simulink model "H8_6GDL_nolineal_desactualizado"  (R2022b)
settings: Solver=VariableStepAuto  StartTime=0.0  StopTime=3  MaxStep=1e-3  RelTol=1e-3
InitFcn:
  | %load("ems.mat");
  | %load("hems.mat");
  | %load("Ka.mat");
  | load('fuerzasY_LIM.mat')
  | load('matrices_linealizacion_6gdl.mat')
  | m = 200;
  | g = 9.81;
  | 
  | x_lev12 = 0.443;
  | x_lev34 = 0.542;%0.443;
  | x_guid12 = 0.4475;
  | x_guid34 = 0.5465;
  | x_lim = 0.0495;
  | 
  | y_lev13 = 0.23686;
  | y_lev24 = 0.23686;
  | y_guid13 = 0.24263;
  | y_guid24 = 0.24263;
  | y_lim = 0.0005;
  | y_brk = 0.21552;
  | 
  | z_lev = 0.08546;
  | z_guid = 0.026;
  | z_lim = 0.1055;
  | z_brk = 0.03941;
  | 
  | kp_lev = 50;
  | ki_lev = 400;
  | kp_guid = 6;
  | ki_guid = 46.5;
  | 
  | Imax_lev = 50;
  | Imin_lev = -50;
  | Imax_guid = 50;
  | Imin_guid = 0;
  | 
  | cg_nom=0.567;
  | lev_nom=0.01965;
  | cg_suelo=0.56985;
  | cg_techo=0.55735;
  | 
  | I = [43.082 0 0; 0 26.887 -0; 0 0 29.297]
values from neighbouring files (symbols this model uses):
  A6 = [0 0 0 0 0 0 0 0 0 0 0 0 ... (100 elements, 10x10)]    [matrices_linealizacion_6gdl.mat]
  B6 = [0 0 0 0 0 0.000575563603666 -0.0459993641186 -0.0505103975277 0.151580453785 0.00175830093621 0 0 ... (80 elements, 10x8)]    [matrices_linealizacion_6gdl.mat]
  C6 = [1 0 0 0 0 0 0 0 0 0 0 1 ... (100 elements, 10x10)]    [matrices_linealizacion_6gdl.mat]
  current = [0 10 20 30 40 50 60 70 80 90 100]    [fuerzasY_LIM.mat]
  D6 = [0 0 0 0 0 0 0 0 0 0 0 0 ... (80 elements, 10x8)]    [matrices_linealizacion_6gdl.mat]
  Ka = [34.5916764023 4.46928641015 34.7816336405 4.65924364837 92.2484067139 -92.2484067139 74.2332308826 -74.2332308826 -4220.94514487 -4209.6309051 -4205.06787146 -4193.7536317 ... (120 elements, 8x15)]    [Ka.mat]    (also in linealizacion_5gdl_bien.m = place(Aa,Ba,[ -1.5 -1.5 -1.5 -1.5 -2 -2 -6 -6 -7 -7 -5 -5 -2; linealizacion_EMS.m = place(Aa,Ba,[ -1 -1 -2 -2 -3 -3 -6 -6 -7 -7 -5 -5 -4 -4 -5 -)
  Y = [0 1 2 3 4 5 6]    [fuerzasY_LIM.mat]
undefined symbols (not defined in the file or in its folder): ems, FuerzaRail_Y, hems, magnitude
libraries: slpidlib x16
(part 1 of 2)
settings Model: Creator=USUARIO  LastModifiedBy=USUARIO
settings SolverCC: ZeroCrossAlgorithm=Adaptive

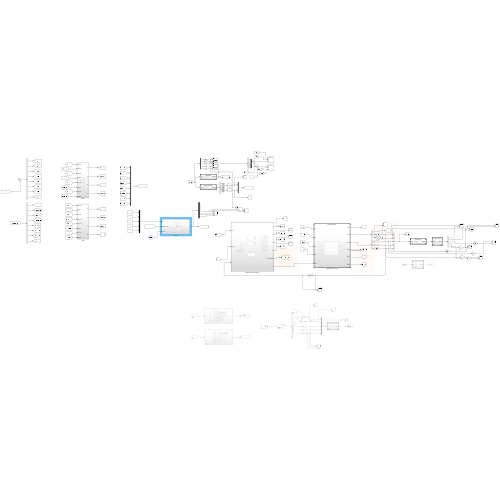
[thumbnail: Simulink's stored preview of the top-level diagram]
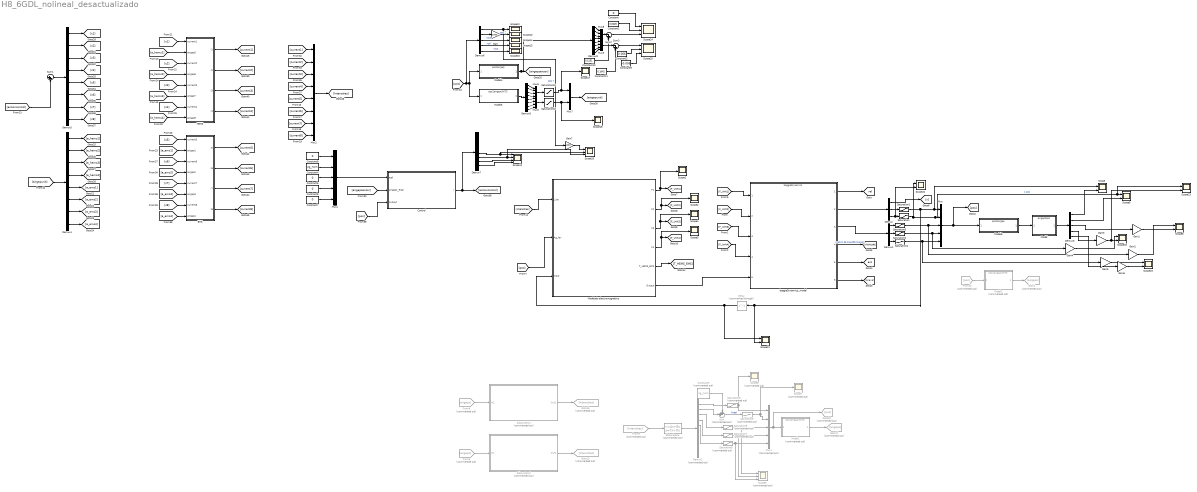
== system H8_6GDL_nolineal_desactualizado ==
  Constant{,5..8} (5 alike) : Constant  Value=0
  Constant1 : Constant  Value=0.0225
  Constant10 : Constant  Value=0.1251
  Constant11 : Constant  Value=0.1042
  Constant2 : Constant  Value=0.006
  Constant3 : Constant  Commented=on  Value=cg_nom
  Constant4 : Constant  Value=cg_nom
  Constant9 : Constant  Value=-0.006
  Control : Subsystem
  Delay : Delay  Commented=through  DelayLength=1  InitialCondition=0.001
  Demux : Demux  Outputs=3
  Demux1 : Demux  Outputs=3
  Demux2 : Demux  Commented=on  Outputs=10
      settings: DisplayOption=none
  Demux3 : Demux  Outputs=5
  Demux{4..5,7..9} (5 alike) : Demux  Outputs=8
  Demux6 : Demux  Outputs=5
  EMS : Subsystem
  From40 : From  Commented=on  GotoTag=pos
  From6 : From  Commented=on  GotoTag=airgaps
  From8 : From  Commented=on  GotoTag=airgaps
  From9 : From  Commented=on  GotoTag=Intensities
  Gain : Gain  Gain=1000
  Gain{1..6} (6 alike) : Gain  Gain=180/pi
  Gain7 : Gain  Gain=1000
  Goto1 : Goto  Commented=on  GotoTag=airgaps
  Goto13 : Goto  Commented=on  GotoTag=Intensities
  Goto16 : Goto  Commented=on  GotoTag=Intensities
  Goto17 : Goto  Commented=on  GotoTag=airgaps
  Goto18 : Goto  Commented=on  GotoTag=pos
  HEMS : Subsystem
  Model : ModelReference  ModelNameDialog=airgap2pos.slx  SimulationMode=Normal  ModelReferenceVersion=1.7
  Model1 : ModelReference  Commented=on  ModelNameDialog=pos2airgapUNITS.slx  SimulationMode=Normal  ModelReferenceVersion=1.3
  Model2 : ModelReference  Commented=on  ModelNameDialog=pos2airgapUNITS.slx  SimulationMode=Normal  ModelReferenceVersion=1.3
  Model4 : ModelReference  ModelNameDialog=pos2airgap.slx  SimulationMode=Normal  ModelReferenceVersion=1.6
  Model5 : ModelReference  ModelNameDialog=pos2airgapUNITS.slx  SimulationMode=Normal  ModelReferenceVersion=1.3
  Model6 : ModelReference  ModelNameDialog=pos2airgap.slx  SimulationMode=Normal  ModelReferenceVersion=1.6
  Modelado electromagnetico : Subsystem
  Mux : Mux  Inputs=5
  Mux1 : Mux  Commented=on  Inputs=5
  Mux2 : Mux  Inputs=8
  Mux{3,5..6,8} (4 alike) : Mux
  Mux4 : Mux  Inputs=5
  Mux7 : Mux  Inputs=2
  Saturation : Saturate  UpperLimit=cg_suelo  LowerLimit=cg_techo
  Saturation1 : Saturate  UpperLimit=0.012  LowerLimit=-0.012
  Saturation15 : Saturate  UpperLimit=0.0225  LowerLimit=0.01
  Saturation16 : Saturate  UpperLimit=0.024  LowerLimit=0
  Saturation2 : Saturate  UpperLimit=0.01268  LowerLimit=-0.01268
  Saturation3 : Saturate  UpperLimit=0.0476  LowerLimit=-0.0476
  Saturation4 : Saturate  UpperLimit=0.024  LowerLimit=-0.024
  Saturation5 : Saturate  Commented=on  UpperLimit=cg_suelo  LowerLimit=cg_techo
  Saturation6 : Saturate  Commented=on  UpperLimit=0.012  LowerLimit=-0.012
  Saturation7 : Saturate  Commented=on  UpperLimit=0.01268  LowerLimit=-0.01268
  Saturation8 : Saturate  Commented=on  UpperLimit=0.0476  LowerLimit=-0.0476
  Saturation9 : Saturate  Commented=on  UpperLimit=0.024  LowerLimit=-0.024
  Scope{,5..6,18..19,21..23} (8 alike) : Scope  NumInputPorts=2
  Scope{1..4,10,12..17} (11 alike) : Scope
  Scope11 : Scope  NumInputPorts=4
  Scope20 : Scope  NumInputPorts=3
  Scope24 : Scope  NumInputPorts=3
  Scope25 : Scope  NumInputPorts=3
  Scope7 : Scope  Commented=on
  Scope8 : Scope  Commented=on
  Scope9 : Scope  Commented=on  NumInputPorts=3
  State-Space : StateSpace  Commented=on  A=A6  B=B6  C=C6  D=D6  InitialCondition=[-0.001 0.001 0.001 -0.001 0.001 0 0 0 0 0]
  Subsystem1 : Subsystem  Commented=on
  Subsystem2 : Subsystem  Commented=on
  Sum : Sum  Commented=on  Inputs=++|
  Sum1 : Sum  Inputs=|+-
  Sum2 : Sum  Inputs=|-+
  Sum3 : Sum  Inputs=|-+
  boggieDynamics_model : ModelReference  ModelNameDialog=boggieDynamics.mdl  SimulationMode=Normal  ModelReferenceVersion=1.35
  tag scope: acc=global, vel=global
  wires:
  [F_Unit4] -> boggieDynamics_model/4
  [F_Unit3] -> boggieDynamics_model/3
  [F_Unit2] -> boggieDynamics_model/2
  boggieDynamics_model/4 -> [Attitude]  "matriz de transformacion"
  [F_Unit1] -> boggieDynamics_model/1
  boggieDynamics_model/3 -> Demux1/1
  Mux/1 -> Model6/1, [pos]
  boggieDynamics_model/2 -> Demux/1
  Demux/3 -> Scope22/2, Saturation/1
  Demux/1 -> [x]
  boggieDynamics_model/1 -> [vel]
  Demux/2 -> Saturation1/1
  boggieDynamics_model/5 -> [acc]
  boggieDynamics_model/6 -> [angvel]
  [pos] -> Modelado electromagnetico/2(Ag_lev)
  [Intensities] -> Modelado electromagnetico/1(I_lev)
  Modelado electromagnetico/3(F3) -> Scope4/1, [F_Unit3]
  Modelado electromagnetico/2(F2) -> Scope2/1, [F_Unit2]
  Modelado electromagnetico/1(F1) -> Scope1/1, [F_Unit1]
  Modelado electromagnetico/5(T_HEMS_EMS) -> [T_HEMS_EMS]
  Demux1/1 -> Saturation3/1
  Demux1/2 -> Saturation2/1
  Demux1/3 -> Saturation4/1
  Model2/1 -> Goto1/1
  Saturation1/1 -> Scope21/2, Delay/1, Scope/1, Mux/1
  Saturation/1 -> Scope22/1, Scope23/1, Scope5/1, Mux/2  "z pos"
  Saturation3/1 -> Gain2/1, Mux/3
  Saturation2/1 -> Gain4/1, Mux/4
  Saturation4/1 -> Gain5/1, Mux/5
  Modelado electromagnetico/4(F4) -> Scope3/1, [F_Unit4]
  Subsystem1/1(Out1) -> Goto16/1
  From8/1 -> Subsystem1/1(In1)
  From6/1 -> Subsystem2/1(In1)
  Subsystem2/1(Out1) -> Goto13/1
  From9/1 -> State-Space/1
  State-Space/1 -> Demux2/1
  Demux2/3 -> Saturation8/1
  Saturation7/1 -> Scope9/2, Mux1/4
  Saturation8/1 -> Mux1/3, Scope9/1
  Demux2/4 -> Saturation7/1
  Saturation9/1 -> Mux1/5, Scope9/3
  Model1/1 -> Goto17/1
  Demux2/5 -> Saturation9/1
  Saturation6/1 -> Mux1/1, Scope8/1
  Demux2/1 -> Saturation6/1
  Mux1/1 -> Model1/1, Goto18/1
  Constant3/1 -> Sum/1
  Demux2/2 -> Sum/2
  Sum/1 -> Saturation5/1  "lineal"
  Saturation5/1 -> Mux1/2, Scope7/1
  Demux4/5 -> [a_ems1]
  HEMS/2(I2) -> [current2]
  [a_hems1] -> HEMS/2(airgap5)
  Demux4/7 -> [a_ems3]
  [current8] -> Mux2/8
  Demux4/8 -> [a_ems4]
  Demux5/5 -> [c5]
  Demux4/6 -> [a_ems2]
  [accioncontrol] -> Sum1/2
  [airgapsensor] -> Control/2(airgaps_Real)
  Demux4/2 -> [a_hems2]
  Demux5/2 -> [c2]
  Demux5/4 -> [c4]
  Mux7/1 -> [airgapunit]
  Saturation16/1 -> Scope16/1, Mux7/2
  Saturation15/1 -> Scope17/1, Mux7/1
  Demux7/8 -> Scope11/4
  Mux5/1 -> Saturation16/1
  Demux8/6 -> Mux5/2
  Demux8/7 -> Mux5/3
  Mux6/1 -> Saturation15/1
  Demux8/3 -> Mux6/3
  Demux8/5 -> Mux5/1
  Demux5/3 -> [c3]
  Demux8/2 -> Mux6/2
  Sum1/1 -> Demux5/1
  [current5] -> Mux2/5
  Demux6/3 -> Scope14/1  "rotX"
  [current6] -> Mux2/6
  [current7] -> Mux2/7
  HEMS/1(I1) -> [current1]
  Demux7/5 -> Scope20/2, Scope11/1
  Constant5/1 -> Mux4/3
  [a_ems1] -> EMS/2(airgap1)
  Mux4/1 -> Control/1(Ref)
  [c8] -> EMS/7(current8)
  [c3] -> HEMS/5(current3)
  Demux6/5 -> Scope15/1  "rotZ"
  Demux5/1 -> [c1]
  [c5] -> EMS/1(current5)
  Demux7/6 -> Scope20/3, Scope11/2
  Constant6/1 -> Mux4/4
  [c2] -> HEMS/3(current2)
  [current1] -> Mux2/1
  [c1] -> HEMS/1(current1)
  [a_hems3] -> HEMS/6(airgap7)
  [a_ems3] -> EMS/6(airgap3)
  [a_hems4] -> HEMS/8(airgap8)
  Demux4/1 -> [a_hems1]
  [a_ems4] -> EMS/8(airgap4)
  [a_hems2] -> HEMS/4(airgap6)
  Demux5/7 -> [c7]
  [current3] -> Mux2/3
  Model4/1 -> Demux9/1, [airgapsensor]
  [c4] -> HEMS/7(current4)
  [c7] -> EMS/5(current7)
  Demux6/4 -> Scope13/1  "rotY"
  Demux7/7 -> Scope11/3
  Demux4/4 -> [a_hems4]
  EMS/4(I8) -> [current8]
  EMS/2(I6) -> [current6]
  Gain/1 -> Scope10/1  "pos Z"
  Constant4/1 -> Mux4/2
  Constant8/1 -> Mux4/1
  Demux5/6 -> [c6]
  Constant7/1 -> Mux4/5
  Demux4/3 -> [a_hems3]
  Demux8/8 -> Mux5/4
  Demux6/2 -> Gain/1
  EMS/3(I7) -> [current7]
  Demux8/1 -> Mux6/1
  [current2] -> Mux2/2
  [a_ems2] -> EMS/4(airgap2)
  [current4] -> Mux2/4
  Demux5/8 -> [c8]
  Mux2/1 -> [Intensities]
  Demux6/1 -> Gain7/1, Scope12/1  "pos Y"
  [c6] -> EMS/3(current6)
  Demux8/4 -> Mux6/4
  HEMS/3(I3) -> [current3]
  HEMS/4(I4) -> [current4]
  [airgapunit] -> Demux4/1
  EMS/1(I5) -> [current5]
  [pos] -> Demux6/1, Model4/1, Model5/1
  Model5/1 -> Demux8/1
  Control/1(I) -> Demux7/1, [accioncontrol]
  [pos] -> Control/3(Output)
  From40/1 -> Model2/1
  Model6/1 -> Model/1
  Model/1 -> Demux3/1
  Demux3/1 -> Scope/2
  Demux3/2 -> Scope5/2
  Demux3/3 -> Gain1/1
  Demux3/4 -> Gain3/1
  Demux3/5 -> Gain6/1
  Modelado electromagnetico/6(Output) -> boggieDynamics_model/5
  Delay/1 -> Scope21/1, Modelado electromagnetico/3(Input)
  Gain1/1 -> Scope6/2
  Gain2/1 -> Scope6/1
  Gain3/1 -> Scope23/2, Scope18/2
  Gain4/1 -> Scope18/1
  Gain5/1 -> Scope19/1
  Gain6/1 -> Scope19/2
  Gain7/1 -> Scope20/1
  Demux9/6 -> Mux3/2
  Demux9/8 -> Mux3/4
  Demux9/4 -> Mux8/4
  Demux9/7 -> Mux3/3
  Demux9/5 -> Mux3/1
  Demux9/3 -> Mux8/3
  Demux9/1 -> Mux8/1
  Mux3/1 -> Sum3/1
  Mux8/1 -> Sum2/1
  Demux9/2 -> Mux8/2
  Sum2/1 -> Scope24/3
  Constant1/1 -> Scope24/2
  Constant/1 -> Scope24/1
  Sum3/1 -> Scope25/1
  Constant9/1 -> Scope25/3
  Constant2/1 -> Scope25/2
  Constant10/1 -> Sum2/2
  Constant11/1 -> Sum3/2

== system H8_6GDL_nolineal_desactualizado/Control ==
  Ref : Inport
  airgaps_Real : Inport  Port=2
  Output : Inport  Port=3
  Demux : Demux  Outputs=5
  Demux1 : Demux  Outputs=5
  Model : ModelReference  ModelNameDialog=airgap2pos.slx  SimulationMode=Normal  ModelReferenceVersion=1.7
  Saturation4 : Saturate  Commented=through  UpperLimit=55  LowerLimit=-55
  Scope{,1..4} (5 alike) : Scope  NumInputPorts=2
  state space control : Subsystem
  I : Outport
  wires:
  airgaps_Real/1 -> Model/1
  Saturation4/1 -> I/1
  Model/1 -> Demux/1
  Ref/1 -> state space control/2(In2)
  state space control/1(Out1) -> Saturation4/1
  Demux/1 -> Scope1/1
  Demux/3 -> Scope/1
  Demux/4 -> Scope3/2
  Demux/2 -> Scope2/2
  Output/1 -> state space control/1(Output), Demux1/1
  Demux1/1 -> Scope1/2
  Demux1/2 -> Scope2/1
  Demux1/3 -> Scope/2
  Demux1/4 -> Scope3/1
  Demux1/5 -> Scope4/1
  Demux/5 -> Scope4/2

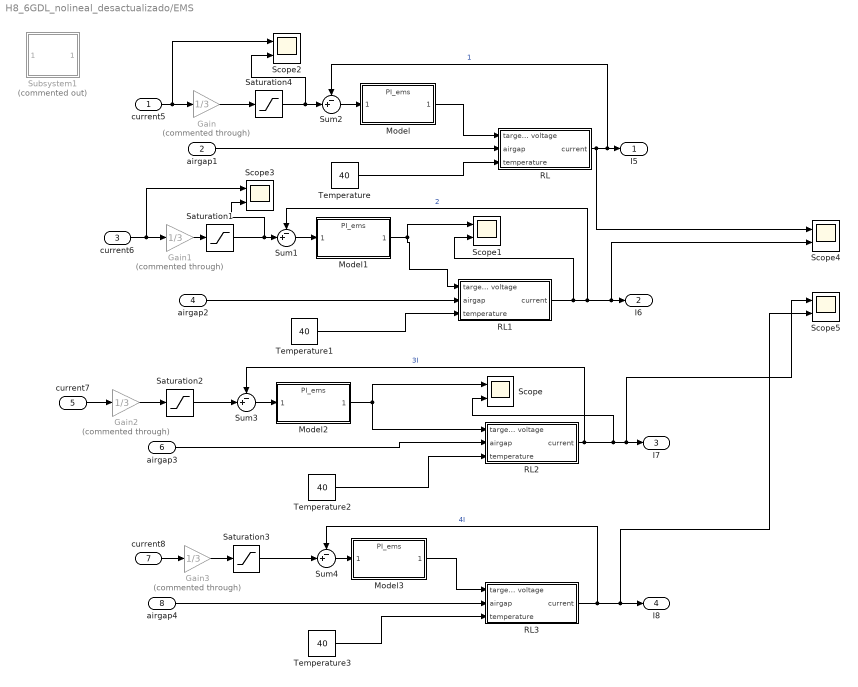
== system H8_6GDL_nolineal_desactualizado/EMS ==
  current5 : Inport
  airgap1 : Inport  Port=2
  current6 : Inport  Port=3
  airgap2 : Inport  Port=4
  current7 : Inport  Port=5
  airgap3 : Inport  Port=6
  current8 : Inport  Port=7
  airgap4 : Inport  Port=8
  Gain{,1..3} (4 alike) : Gain  Commented=through  Gain=1/3
  Model{,1..3} (4 alike) : ModelReference  ModelNameDialog=PI_ems.slx  SimulationMode=Normal  ModelReferenceVersion=1.2
  RL : Subsystem
  RL1 : Subsystem
  RL2 : Subsystem
  RL3 : Subsystem
  Saturation{1..4} (4 alike) : Saturate  UpperLimit=50  LowerLimit=0
  Scope{,1..5} (6 alike) : Scope  NumInputPorts=2
  Subsystem1 : Subsystem  Commented=on
  Sum{1..4} (4 alike) : Sum  Inputs=-+|
  Temperature{,1..3} (4 alike) : Constant  Value=40
  I5 : Outport
  I6 : Outport  Port=2
  I7 : Outport  Port=3
  I8 : Outport  Port=4
  wires:
  Temperature/1 -> RL/3(temperature)
  airgap1/1 -> RL/2(airgap)
  Temperature3/1 -> RL3/3(temperature)
  RL/1(current) -> Scope4/1, I5/1, Sum2/1  "1"
  current8/1 -> Gain3/1
  Temperature1/1 -> RL1/3(temperature)
  Temperature2/1 -> RL2/3(temperature)
  RL3/1(current) -> Scope5/2, I8/1, Sum4/1  "4I"
  current7/1 -> Gain2/1
  airgap2/1 -> RL1/2(airgap)
  RL1/1(current) -> Scope1/2, Scope4/2, I6/1, Sum1/1  "2"
  RL2/1(current) -> Scope/2, Scope5/1, I7/1, Sum3/1  "3I"
  airgap3/1 -> RL2/2(airgap)
  airgap4/1 -> RL3/2(airgap)
  Sum2/1 -> Model/1
  Sum1/1 -> Model1/1
  Sum3/1 -> Model2/1
  Sum4/1 -> Model3/1
  Model/1 -> RL/1(target voltage)
  Model3/1 -> RL3/1(target voltage)
  Model2/1 -> RL2/1(target voltage), Scope/1
  Model1/1 -> RL1/1(target voltage), Scope1/1
  current5/1 -> Scope2/1, Gain/1
  Saturation4/1 -> Scope2/2, Sum2/2
  Saturation1/1 -> Scope3/2, Sum1/2
  Saturation2/1 -> Sum3/2
  Saturation3/1 -> Sum4/2
  current6/1 -> Scope3/1, Gain1/1
  Gain/1 -> Saturation4/1
  Gain1/1 -> Saturation1/1
  Gain2/1 -> Saturation2/1
  Gain3/1 -> Saturation3/1

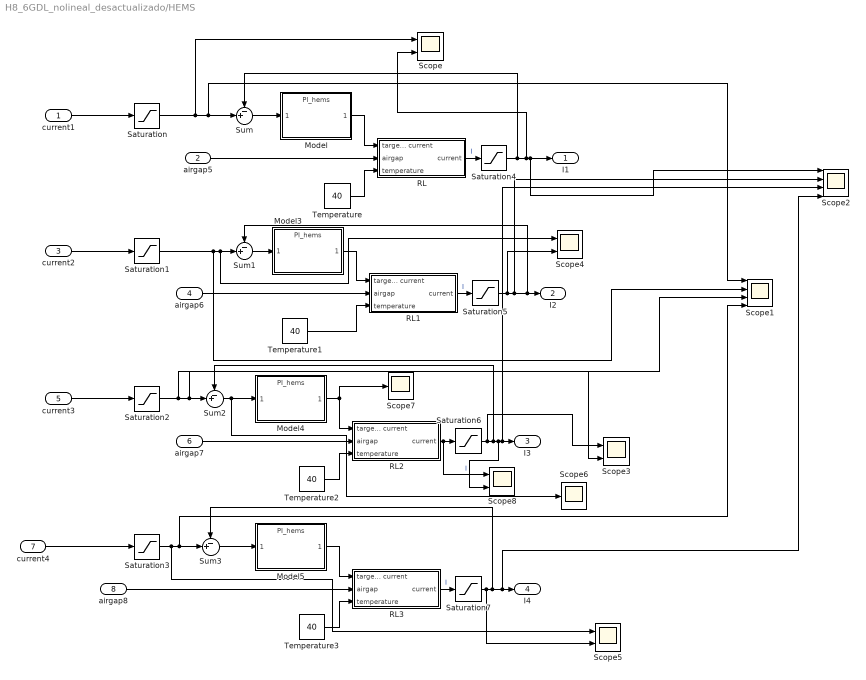
== system H8_6GDL_nolineal_desactualizado/HEMS ==
  current1 : Inport
  airgap5 : Inport  Port=2
  current2 : Inport  Port=3
  airgap6 : Inport  Port=4
  current3 : Inport  Port=5
  airgap7 : Inport  Port=6
  current4 : Inport  Port=7
  airgap8 : Inport  Port=8
  Model{,3..5} (4 alike) : ModelReference  ModelNameDialog=PI_hems.slx  SimulationMode=Normal  ModelReferenceVersion=1.3
  RL : Subsystem
  RL1 : Subsystem
  RL2 : Subsystem
  RL3 : Subsystem
  Saturation{,1..7} (8 alike) : Saturate  UpperLimit=50  LowerLimit=-50
  Scope{,3..5,8} (5 alike) : Scope  NumInputPorts=2
  Scope1 : Scope  NumInputPorts=4
  Scope2 : Scope  NumInputPorts=4
  Scope6 : Scope
  Scope7 : Scope
  Sum{,1..3} (4 alike) : Sum  Inputs=-+|
  Temperature{,1..3} (4 alike) : Constant  Value=40
  I1 : Outport
  I2 : Outport  Port=2
  I3 : Outport  Port=3
  I4 : Outport  Port=4
  wires:
  Temperature/1 -> RL/3(temperature)
  Model3/1 -> RL1/1(target current)
  Model5/1 -> RL3/1(target current)
  Model/1 -> RL/1(target current)
  airgap5/1 -> RL/2(airgap)
  Temperature3/1 -> RL3/3(temperature)
  RL/1(current) -> Saturation4/1  "I"
  Temperature1/1 -> RL1/3(temperature)
  Temperature2/1 -> RL2/3(temperature)
  Model4/1 -> RL2/1(target current), Scope7/1
  RL3/1(current) -> Saturation7/1  "I"
  airgap6/1 -> RL1/2(airgap)
  RL1/1(current) -> Saturation5/1  "I"
  RL2/1(current) -> Scope8/1, Saturation6/1  "I"
  airgap7/1 -> RL2/2(airgap)
  airgap8/1 -> RL3/2(airgap)
  Sum/1 -> Model/1
  Sum1/1 -> Model3/1
  Sum2/1 -> Scope6/1, Model4/1
  Sum3/1 -> Model5/1
  Saturation2/1 -> Scope3/2, Scope1/3, Sum2/2
  Saturation1/1 -> Scope1/2, Scope4/1, Sum1/2
  Saturation/1 -> Scope/1, Scope1/1, Sum/2
  Saturation3/1 -> Scope5/1, Scope1/4, Sum3/2
  current1/1 -> Saturation/1
  current4/1 -> Saturation3/1
  current3/1 -> Saturation2/1
  current2/1 -> Saturation1/1
  Saturation4/1 -> Scope/2, Scope2/1, I1/1, Sum/1
  Saturation5/1 -> Scope4/2, Scope2/2, Sum1/1, I2/1
  Saturation7/1 -> Scope5/2, Scope2/4, I4/1, Sum3/1
  Saturation6/1 -> Scope3/1, Scope8/2, Scope2/3, I3/1, Sum2/1

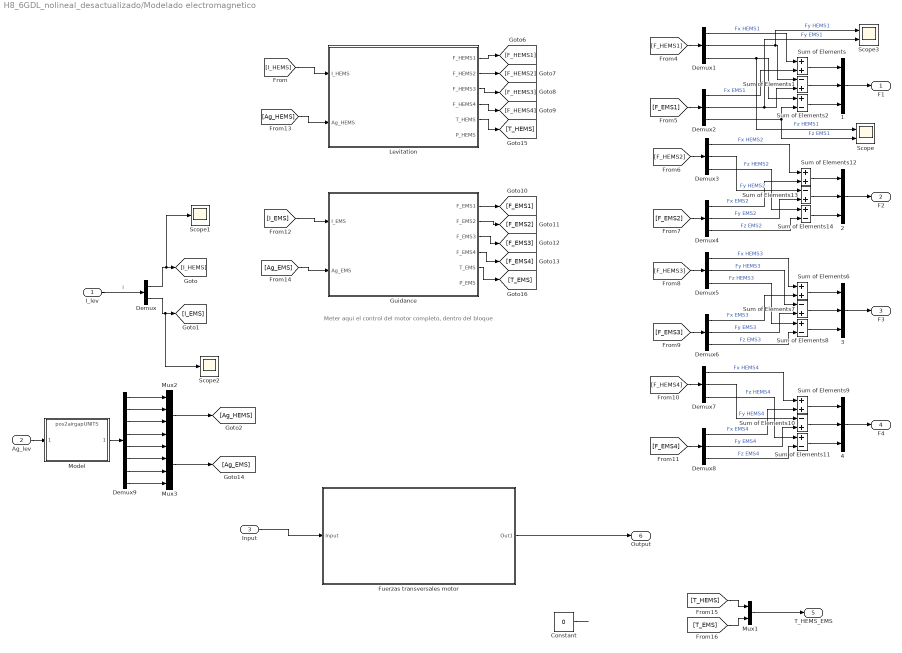
== system H8_6GDL_nolineal_desactualizado/Modelado electromagnetico ==
  note: Meter aqui el control del motor completo, dentro del bloque
  I_lev : Inport
  Ag_lev : Inport  Port=2
  Input : Inport  Port=3
  {1..4} (4 alike) : Mux  Inputs=3
  Constant : Constant  Value=0
  Demux : Demux  Outputs=2
  Demux{1..8} (8 alike) : Demux  Outputs=3
  Demux9 : Demux  Outputs=8
  Fuerzas transversales motor : Subsystem
  Guidance : Subsystem
  Levitation : Subsystem
  Model : ModelReference  ModelNameDialog=pos2airgapUNITS.slx  SimulationMode=Normal  ModelReferenceVersion=1.3
  Mux1 : Mux  Inputs=2
  Mux2 : Mux
  Mux3 : Mux
  Scope : Scope  NumInputPorts=2
  Scope1 : Scope
  Scope2 : Scope
  Scope3 : Scope  NumInputPorts=2
  Sum of Elements{,6,9,12} (4 alike) : Sum
  Sum of Elements{1,7,10,13} (4 alike) : Sum  Inputs=-+
  Sum of Elements{2,8,11,14} (4 alike) : Sum  Inputs=+-
  F1 : Outport
  F2 : Outport  Port=2
  F3 : Outport  Port=3
  F4 : Outport  Port=4
  T_HEMS_EMS : Outport  Port=5
  Output : Outport  Port=6
  wires:
  I_lev/1 -> Demux/1  "I"
  Demux/1 -> Scope1/1, [I_HEMS]
  Demux/2 -> Scope2/1, [I_EMS]
  [I_HEMS] -> Levitation/1(I_HEMS)
  Levitation/1(F_HEMS1) -> [F_HEMS1]
  Levitation/2(F_HEMS2) -> [F_HEMS2]
  Levitation/3(F_HEMS3) -> [F_HEMS3]
  Levitation/4(F_HEMS4) -> [F_HEMS4]
  Sum of Elements/1 -> 1/1
  1/1 -> F1/1
  Sum of Elements1/1 -> 1/2
  Sum of Elements2/1 -> 1/3
  2/1 -> F2/1
  [F_HEMS1] -> Demux1/1
  Demux1/1 -> Sum of Elements/1  "Fx HEMS1"
  Demux1/2 -> Scope3/1, Sum of Elements1/1  "Fy HEMS1"
  Demux1/3 -> Scope/1, Sum of Elements2/1  "Fz HEMS1"
  3/1 -> F3/1
  Sum of Elements8/1 -> 3/3
  Sum of Elements6/1 -> 3/1
  Sum of Elements7/1 -> 3/2
  4/1 -> F4/1
  Sum of Elements11/1 -> 4/3
  Sum of Elements9/1 -> 4/1
  Sum of Elements10/1 -> 4/2
  Guidance/2(F_EMS2) -> [F_EMS2]
  Guidance/3(F_EMS3) -> [F_EMS3]
  Guidance/4(F_EMS4) -> [F_EMS4]
  Guidance/1(F_EMS1) -> [F_EMS1]
  Demux2/1 -> Sum of Elements/2  "Fx EMS1"
  [F_EMS1] -> Demux2/1
  Demux2/2 -> Scope3/2, Sum of Elements1/2  "Fy EMS1"
  Demux2/3 -> Sum of Elements2/2, Scope/2  "Fz EMS1"
  [F_EMS2] -> Demux4/1
  Demux4/1 -> Sum of Elements12/2  "Fx EMS2"
  Demux4/2 -> Sum of Elements13/2  "Fy EMS2"
  Sum of Elements14/1 -> 2/3
  Demux3/1 -> Sum of Elements12/1  "Fx HEMS2"
  [F_HEMS2] -> Demux3/1
  Demux3/2 -> Sum of Elements13/1  "Fy HEMS2"
  Demux3/3 -> Sum of Elements14/1  "Fz HEMS2"
  Sum of Elements13/1 -> 2/2
  Sum of Elements12/1 -> 2/1
  Demux4/3 -> Sum of Elements14/2  "Fz EMS2"
  Demux5/3 -> Sum of Elements8/1  "Fz HEMS3"
  Demux5/2 -> Sum of Elements7/1  "Fy HEMS3"
  [F_HEMS3] -> Demux5/1
  Demux6/3 -> Sum of Elements8/2  "Fz EMS3"
  [F_EMS3] -> Demux6/1
  Demux6/1 -> Sum of Elements6/2  "Fx EMS3"
  Demux5/1 -> Sum of Elements6/1  "Fx HEMS3"
  Demux6/2 -> Sum of Elements7/2  "Fy EMS3"
  Demux7/3 -> Sum of Elements11/1  "Fz HEMS4"
  Demux8/3 -> Sum of Elements11/2  "Fz EMS4"
  Demux8/2 -> Sum of Elements10/2  "Fy EMS4"
  Demux7/2 -> Sum of Elements10/1  "Fy HEMS4"
  Demux7/1 -> Sum of Elements9/1  "Fx HEMS4"
  Demux8/1 -> Sum of Elements9/2  "Fx EMS4"
  [F_HEMS4] -> Demux7/1
  [F_EMS4] -> Demux8/1
  [I_EMS] -> Guidance/1(I_EMS)
  Ag_lev/1 -> Model/1
  [Ag_HEMS] -> Levitation/2(Ag_HEMS)
  [Ag_EMS] -> Guidance/2(Ag_EMS)
  Levitation/5(T_HEMS) -> [T_HEMS]
  Guidance/5(T_EMS) -> [T_EMS]
  Mux1/1 -> T_HEMS_EMS/1
  [T_HEMS] -> Mux1/1
  [T_EMS] -> Mux1/2
  Model/1 -> Demux9/1
  Demux9/1 -> Mux2/1
  Demux9/2 -> Mux2/2
  Demux9/3 -> Mux2/3
  Demux9/4 -> Mux2/4
  Mux2/1 -> [Ag_HEMS]
  Demux9/5 -> Mux3/1
  Demux9/7 -> Mux3/3
  Mux3/1 -> [Ag_EMS]
  Demux9/6 -> Mux3/2
  Demux9/8 -> Mux3/4
  Input/1 -> Fuerzas transversales motor/1(Input)
  Fuerzas transversales motor/1(Out1) -> Output/1
  Constant/1 -> ?

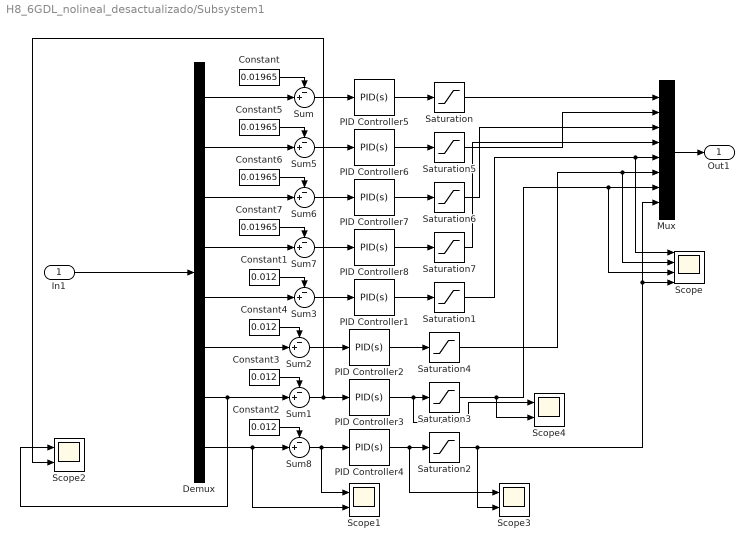
== system H8_6GDL_nolineal_desactualizado/Subsystem1 ==
  In1 : Inport
  Constant{,5..7} (4 alike) : Constant  Value=0.01965
  Constant{1..4} (4 alike) : Constant  Value=0.012
  Demux : Demux  Outputs=8
  Mux : Mux  Inputs=8
  PID Controller{1..4} (4 alike) : slpidlib/PID Controller  Controller=PID  Form=Parallel  TimeDomain=Continuous-time  UseExternalTs=off  SampleTime=-1  IntegratorMethod=Forward Euler  FilterMethod=Forward Euler  ControllerParametersSource=internal  P=6490  I=15500  UseKiTs=off  D=100  N=1900  UseFilter=on  TunerSelectOption=Transfer Function Based (PID Tuner App)  InitialConditionSource=internal  InitialConditionForIntegrator=suelo  InitialConditionForFilter=0  DifferentiatorICPrevScaledInput=0  ExternalReset=none  TrackingMode=off  Kt=1  LimitOutput=off  SatLimitsSource=internal  UpperSaturationLimit=inf  LowerSaturationLimit=-inf  LinearizeAsGain=on  AntiWindupMode=none  Kb=1  LimitIntegrator=off  UpperIntegratorSaturationLimit=inf  LowerIntegratorSaturationLimit=-inf  POutMin=[]  POutMax=[]  IOutMin=[]  IOutMax=[]  DOutMin=[]  DOutMax=[]  NOutMin=[]  NOutMax=[]  SumOutMin=[]  SumOutMax=[]  SaturationOutMin=[]  SaturationOutMax=[]  PParamMin=[]  PParamMax=[]  IParamMin=[]  IParamMax=[]  DParamMin=[]  DParamMax=[]  NParamMin=[]  NParamMax=[]  KbParamMin=[]  KbParamMax=[]  KtParamMin=[]  KtParamMax=[]  KbOutMin=[]  KbOutMax=[]  KtOutMin=[]  KtOutMax=[]  IntegratorOutMin=[]  IntegratorOutMax=[]  FilterOutMin=[]  FilterOutMax=[]  SumI1OutMin=[]  SumI1OutMax=[]  SumI2OutMin=[]  SumI2OutMax=[]  SumI3OutMin=[]  SumI3OutMax=[]  SumI4OutMin=[]  SumI4OutMax=[]  SumDOutMin=[]  SumDOutMax=[]  DifferentiatorOutMin=[]  DifferentiatorOutMax=[]  FilterDiffOutCoefMin=[]  FilterDiffOutCoefMax=[]  ReciprocalOutMin=[]  ReciprocalOutMax=[]  SumDenOutMin=[]  SumDenOutMax=[]  SumNumOutMin=[]  SumNumOutMax=[]  DivideOutMin=[]  DivideOutMax=[]  UdiffTsProdOutMin=[]  UdiffTsProdOutMax=[]  NTsProdOutMin=[]  NTsProdOutMax=[]  UintegralTsProdOutMin=[]  UintegralTsProdOutMax=[]  UngainTsProdOutMin=[]  UngainTsProdOutMax=[]  ClampingZeroOutDataTypeStr=Inherit: Inherit via back propagation  ClampingZeroOutMin=[]  ClampingZeroOutMax=[]  FilterDenConstantOutDataTypeStr=Inherit: Inherit via back propagation  FilterDenConstantOutMin=[]  FilterDenConstantOutMax=[]  PCopyOutDataTypeStr=Inherit: Inherit via back propagation  PCopyOutMin=[]  PCopyOutMax=[]  NCopyOutDataTypeStr=Inherit: Inherit via back propagation  NCopyOutMin=[]  NCopyOutMax=[]  IntegratorContinuousStateAttributes=''  IntegratorStateMustResolveToSignalObject=off  IntegratorRTWStateStorageClass=Auto  FilterContinuousStateAttributes=''  FilterStateMustResolveToSignalObject=off  FilterRTWStateStorageClass=Auto  ParallelPVariant=InternalParameters  IdealPVariant=Disabled  IVariant=InternalParameters  DVariant=InternalParameters  IntegratorVariant=Continuous  SatVariant=Disabled  AWVariant=Passthrough  PCopyVariant=Disabled  TRVariant=Disabled  FdbkBlocksVariant=Forward  IdealPFdbkVariant=Disabled  SatFdbkVariant=Disabled  DerivativeFilterVariant=ContFilter  NVariant=InternalParameters  NCopyVariant=Disabled  FilterICVariant=InternalICsFilter  IntegratorICVariant=InternalICs  ExternalResetVariant=Disabled  TRSumVariant=Passthrough  SumFdbkVariant=Disabled  SumVariant=Sum_PID  TsampFilterVariant=InternalTs  TsampNgainVariant=Passthrough  TsampIntegralVariant=Passthrough  ExternalSaturationOutDataTypeStr=Inherit: Same as second input
  PID Controller{5..8} (4 alike) : slpidlib/PID Controller  Controller=PID  Form=Parallel  TimeDomain=Continuous-time  UseExternalTs=off  SampleTime=-1  IntegratorMethod=Forward Euler  FilterMethod=Forward Euler  ControllerParametersSource=internal  P=64900  I=155000  UseKiTs=off  D=1000  N=1900  UseFilter=on  TunerSelectOption=Transfer Function Based (PID Tuner App)  InitialConditionSource=internal  InitialConditionForIntegrator=suelo  InitialConditionForFilter=0  DifferentiatorICPrevScaledInput=0  ExternalReset=none  TrackingMode=off  Kt=1  LimitOutput=off  SatLimitsSource=internal  UpperSaturationLimit=inf  LowerSaturationLimit=-inf  LinearizeAsGain=on  AntiWindupMode=none  Kb=1  LimitIntegrator=off  UpperIntegratorSaturationLimit=inf  LowerIntegratorSaturationLimit=-inf  POutMin=[]  POutMax=[]  IOutMin=[]  IOutMax=[]  DOutMin=[]  DOutMax=[]  NOutMin=[]  NOutMax=[]  SumOutMin=[]  SumOutMax=[]  SaturationOutMin=[]  SaturationOutMax=[]  PParamMin=[]  PParamMax=[]  IParamMin=[]  IParamMax=[]  DParamMin=[]  DParamMax=[]  NParamMin=[]  NParamMax=[]  KbParamMin=[]  KbParamMax=[]  KtParamMin=[]  KtParamMax=[]  KbOutMin=[]  KbOutMax=[]  KtOutMin=[]  KtOutMax=[]  IntegratorOutMin=[]  IntegratorOutMax=[]  FilterOutMin=[]  FilterOutMax=[]  SumI1OutMin=[]  SumI1OutMax=[]  SumI2OutMin=[]  SumI2OutMax=[]  SumI3OutMin=[]  SumI3OutMax=[]  SumI4OutMin=[]  SumI4OutMax=[]  SumDOutMin=[]  SumDOutMax=[]  DifferentiatorOutMin=[]  DifferentiatorOutMax=[]  FilterDiffOutCoefMin=[]  FilterDiffOutCoefMax=[]  ReciprocalOutMin=[]  ReciprocalOutMax=[]  SumDenOutMin=[]  SumDenOutMax=[]  SumNumOutMin=[]  SumNumOutMax=[]  DivideOutMin=[]  DivideOutMax=[]  UdiffTsProdOutMin=[]  UdiffTsProdOutMax=[]  NTsProdOutMin=[]  NTsProdOutMax=[]  UintegralTsProdOutMin=[]  UintegralTsProdOutMax=[]  UngainTsProdOutMin=[]  UngainTsProdOutMax=[]  ClampingZeroOutDataTypeStr=Inherit: Inherit via back propagation  ClampingZeroOutMin=[]  ClampingZeroOutMax=[]  FilterDenConstantOutDataTypeStr=Inherit: Inherit via back propagation  FilterDenConstantOutMin=[]  FilterDenConstantOutMax=[]  PCopyOutDataTypeStr=Inherit: Inherit via back propagation  PCopyOutMin=[]  PCopyOutMax=[]  NCopyOutDataTypeStr=Inherit: Inherit via back propagation  NCopyOutMin=[]  NCopyOutMax=[]  IntegratorContinuousStateAttributes=''  IntegratorStateMustResolveToSignalObject=off  IntegratorRTWStateStorageClass=Auto  FilterContinuousStateAttributes=''  FilterStateMustResolveToSignalObject=off  FilterRTWStateStorageClass=Auto  ParallelPVariant=InternalParameters  IdealPVariant=Disabled  IVariant=InternalParameters  DVariant=InternalParameters  IntegratorVariant=Continuous  SatVariant=Disabled  AWVariant=Passthrough  PCopyVariant=Disabled  TRVariant=Disabled  FdbkBlocksVariant=Forward  IdealPFdbkVariant=Disabled  SatFdbkVariant=Disabled  DerivativeFilterVariant=ContFilter  NVariant=InternalParameters  NCopyVariant=Disabled  FilterICVariant=InternalICsFilter  IntegratorICVariant=InternalICs  ExternalResetVariant=Disabled  TRSumVariant=Passthrough  SumFdbkVariant=Disabled  SumVariant=Sum_PID  TsampFilterVariant=InternalTs  TsampNgainVariant=Passthrough  TsampIntegralVariant=Passthrough  ExternalSaturationOutDataTypeStr=Inherit: Same as second input
  Saturation{,5..7} (4 alike) : Saturate  UpperLimit=50  LowerLimit=-50
  Saturation{1..4} (4 alike) : Saturate  UpperLimit=50  LowerLimit=0
  Scope : Scope  NumInputPorts=4
  Scope{1..4} (4 alike) : Scope  NumInputPorts=2
  Sum{,1..3,5..8} (8 alike) : Sum  Inputs=-+|
  Out1 : Outport
  wires:
  In1/1 -> Demux/1
  Demux/1 -> Sum/2
  Sum/1 -> PID Controller5/1
  Constant/1 -> Sum/1
  PID Controller5/1 -> Saturation/1
  Mux/1 -> Out1/1
  Saturation/1 -> Mux/1
  Saturation1/1 -> Scope/1, Mux/5
  Sum3/1 -> PID Controller1/1
  PID Controller1/1 -> Saturation1/1
  Demux/5 -> Sum3/2
  Constant1/1 -> Sum3/1
  Demux/8 -> Sum8/2, Scope1/2
  PID Controller4/1 -> Scope3/1, Saturation2/1
  Saturation2/1 -> Scope3/2, Scope/4, Mux/8
  Constant2/1 -> Sum8/1
  Demux/7 -> Sum1/2, Scope2/1
  Constant3/1 -> Sum1/1
  PID Controller3/1 -> Scope4/1, Saturation3/1
  Saturation3/1 -> Scope4/2, Scope/3, Mux/7
  Sum1/1 -> PID Controller3/1, Scope2/2
  Demux/6 -> Sum2/2
  Constant4/1 -> Sum2/1
  PID Controller2/1 -> Saturation4/1
  Saturation4/1 -> Scope/2, Mux/6
  Sum2/1 -> PID Controller2/1
  PID Controller6/1 -> Saturation5/1
  Constant5/1 -> Sum5/1
  Demux/2 -> Sum5/2
  Sum5/1 -> PID Controller6/1
  PID Controller7/1 -> Saturation6/1
  Constant6/1 -> Sum6/1
  Saturation6/1 -> Mux/3
  Demux/3 -> Sum6/2
  Sum6/1 -> PID Controller7/1
  Sum7/1 -> PID Controller8/1
  PID Controller8/1 -> Saturation7/1
  Demux/4 -> Sum7/2
  Constant7/1 -> Sum7/1
  Saturation7/1 -> Mux/4
  Saturation5/1 -> Mux/2
  Sum8/1 -> PID Controller4/1, Scope1/1

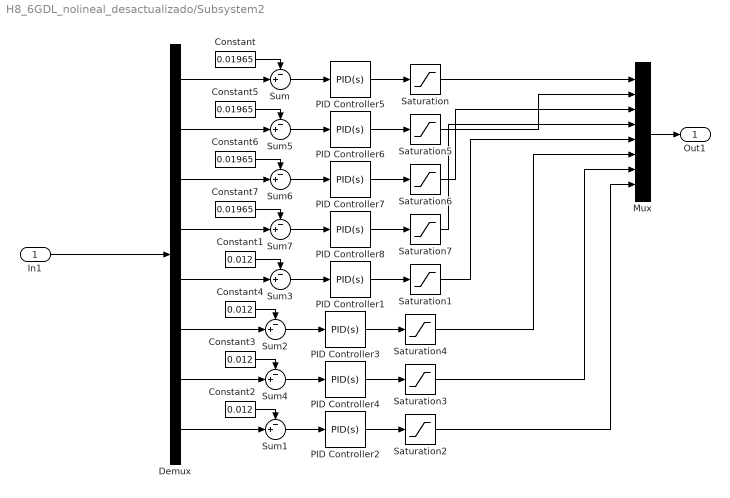
== system H8_6GDL_nolineal_desactualizado/Subsystem2 ==
  In1 : Inport
  Constant{,5..7} (4 alike) : Constant  Value=0.01965
  Constant{1..4} (4 alike) : Constant  Value=0.012
  Demux : Demux  Outputs=8
  Mux : Mux  Inputs=8
  PID Controller{1..4} (4 alike) : slpidlib/PID Controller  Controller=PID  Form=Parallel  TimeDomain=Continuous-time  UseExternalTs=off  SampleTime=-1  IntegratorMethod=Forward Euler  FilterMethod=Forward Euler  ControllerParametersSource=internal  P=5490  I=10500  UseKiTs=off  D=350  N=1900  UseFilter=on  TunerSelectOption=Transfer Function Based (PID Tuner App)  InitialConditionSource=internal  InitialConditionForIntegrator=suelo  InitialConditionForFilter=0  DifferentiatorICPrevScaledInput=0  ExternalReset=none  TrackingMode=off  Kt=1  LimitOutput=off  SatLimitsSource=internal  UpperSaturationLimit=inf  LowerSaturationLimit=-inf  LinearizeAsGain=on  AntiWindupMode=none  Kb=1  LimitIntegrator=off  UpperIntegratorSaturationLimit=inf  LowerIntegratorSaturationLimit=-inf  POutMin=[]  POutMax=[]  IOutMin=[]  IOutMax=[]  DOutMin=[]  DOutMax=[]  NOutMin=[]  NOutMax=[]  SumOutMin=[]  SumOutMax=[]  SaturationOutMin=[]  SaturationOutMax=[]  PParamMin=[]  PParamMax=[]  IParamMin=[]  IParamMax=[]  DParamMin=[]  DParamMax=[]  NParamMin=[]  NParamMax=[]  KbParamMin=[]  KbParamMax=[]  KtParamMin=[]  KtParamMax=[]  KbOutMin=[]  KbOutMax=[]  KtOutMin=[]  KtOutMax=[]  IntegratorOutMin=[]  IntegratorOutMax=[]  FilterOutMin=[]  FilterOutMax=[]  SumI1OutMin=[]  SumI1OutMax=[]  SumI2OutMin=[]  SumI2OutMax=[]  SumI3OutMin=[]  SumI3OutMax=[]  SumI4OutMin=[]  SumI4OutMax=[]  SumDOutMin=[]  SumDOutMax=[]  DifferentiatorOutMin=[]  DifferentiatorOutMax=[]  FilterDiffOutCoefMin=[]  FilterDiffOutCoefMax=[]  ReciprocalOutMin=[]  ReciprocalOutMax=[]  SumDenOutMin=[]  SumDenOutMax=[]  SumNumOutMin=[]  SumNumOutMax=[]  DivideOutMin=[]  DivideOutMax=[]  UdiffTsProdOutMin=[]  UdiffTsProdOutMax=[]  NTsProdOutMin=[]  NTsProdOutMax=[]  UintegralTsProdOutMin=[]  UintegralTsProdOutMax=[]  UngainTsProdOutMin=[]  UngainTsProdOutMax=[]  ClampingZeroOutDataTypeStr=Inherit: Inherit via back propagation  ClampingZeroOutMin=[]  ClampingZeroOutMax=[]  FilterDenConstantOutDataTypeStr=Inherit: Inherit via back propagation  FilterDenConstantOutMin=[]  FilterDenConstantOutMax=[]  PCopyOutDataTypeStr=Inherit: Inherit via back propagation  PCopyOutMin=[]  PCopyOutMax=[]  NCopyOutDataTypeStr=Inherit: Inherit via back propagation  NCopyOutMin=[]  NCopyOutMax=[]  IntegratorContinuousStateAttributes=''  IntegratorStateMustResolveToSignalObject=off  IntegratorRTWStateStorageClass=Auto  FilterContinuousStateAttributes=''  FilterStateMustResolveToSignalObject=off  FilterRTWStateStorageClass=Auto  ParallelPVariant=InternalParameters  IdealPVariant=Disabled  IVariant=InternalParameters  DVariant=InternalParameters  IntegratorVariant=Continuous  SatVariant=Disabled  AWVariant=Passthrough  PCopyVariant=Disabled  TRVariant=Disabled  FdbkBlocksVariant=Forward  IdealPFdbkVariant=Disabled  SatFdbkVariant=Disabled  DerivativeFilterVariant=ContFilter  NVariant=InternalParameters  NCopyVariant=Disabled  FilterICVariant=InternalICsFilter  IntegratorICVariant=InternalICs  ExternalResetVariant=Disabled  TRSumVariant=Passthrough  SumFdbkVariant=Disabled  SumVariant=Sum_PID  TsampFilterVariant=InternalTs  TsampNgainVariant=Passthrough  TsampIntegralVariant=Passthrough  ExternalSaturationOutDataTypeStr=Inherit: Same as second input
  PID Controller{5..8} (4 alike) : slpidlib/PID Controller  Controller=PID  Form=Parallel  TimeDomain=Continuous-time  UseExternalTs=off  SampleTime=-1  IntegratorMethod=Forward Euler  FilterMethod=Forward Euler  ControllerParametersSource=internal  P=64900  I=155000  UseKiTs=off  D=1000  N=1900  UseFilter=on  TunerSelectOption=Transfer Function Based (PID Tuner App)  InitialConditionSource=internal  InitialConditionForIntegrator=suelo  InitialConditionForFilter=0  DifferentiatorICPrevScaledInput=0  ExternalReset=none  TrackingMode=off  Kt=1  LimitOutput=off  SatLimitsSource=internal  UpperSaturationLimit=inf  LowerSaturationLimit=-inf  LinearizeAsGain=on  AntiWindupMode=none  Kb=1  LimitIntegrator=off  UpperIntegratorSaturationLimit=inf  LowerIntegratorSaturationLimit=-inf  POutMin=[]  POutMax=[]  IOutMin=[]  IOutMax=[]  DOutMin=[]  DOutMax=[]  NOutMin=[]  NOutMax=[]  SumOutMin=[]  SumOutMax=[]  SaturationOutMin=[]  SaturationOutMax=[]  PParamMin=[]  PParamMax=[]  IParamMin=[]  IParamMax=[]  DParamMin=[]  DParamMax=[]  NParamMin=[]  NParamMax=[]  KbParamMin=[]  KbParamMax=[]  KtParamMin=[]  KtParamMax=[]  KbOutMin=[]  KbOutMax=[]  KtOutMin=[]  KtOutMax=[]  IntegratorOutMin=[]  IntegratorOutMax=[]  FilterOutMin=[]  FilterOutMax=[]  SumI1OutMin=[]  SumI1OutMax=[]  SumI2OutMin=[]  SumI2OutMax=[]  SumI3OutMin=[]  SumI3OutMax=[]  SumI4OutMin=[]  SumI4OutMax=[]  SumDOutMin=[]  SumDOutMax=[]  DifferentiatorOutMin=[]  DifferentiatorOutMax=[]  FilterDiffOutCoefMin=[]  FilterDiffOutCoefMax=[]  ReciprocalOutMin=[]  ReciprocalOutMax=[]  SumDenOutMin=[]  SumDenOutMax=[]  SumNumOutMin=[]  SumNumOutMax=[]  DivideOutMin=[]  DivideOutMax=[]  UdiffTsProdOutMin=[]  UdiffTsProdOutMax=[]  NTsProdOutMin=[]  NTsProdOutMax=[]  UintegralTsProdOutMin=[]  UintegralTsProdOutMax=[]  UngainTsProdOutMin=[]  UngainTsProdOutMax=[]  ClampingZeroOutDataTypeStr=Inherit: Inherit via back propagation  ClampingZeroOutMin=[]  ClampingZeroOutMax=[]  FilterDenConstantOutDataTypeStr=Inherit: Inherit via back propagation  FilterDenConstantOutMin=[]  FilterDenConstantOutMax=[]  PCopyOutDataTypeStr=Inherit: Inherit via back propagation  PCopyOutMin=[]  PCopyOutMax=[]  NCopyOutDataTypeStr=Inherit: Inherit via back propagation  NCopyOutMin=[]  NCopyOutMax=[]  IntegratorContinuousStateAttributes=''  IntegratorStateMustResolveToSignalObject=off  IntegratorRTWStateStorageClass=Auto  FilterContinuousStateAttributes=''  FilterStateMustResolveToSignalObject=off  FilterRTWStateStorageClass=Auto  ParallelPVariant=InternalParameters  IdealPVariant=Disabled  IVariant=InternalParameters  DVariant=InternalParameters  IntegratorVariant=Continuous  SatVariant=Disabled  AWVariant=Passthrough  PCopyVariant=Disabled  TRVariant=Disabled  FdbkBlocksVariant=Forward  IdealPFdbkVariant=Disabled  SatFdbkVariant=Disabled  DerivativeFilterVariant=ContFilter  NVariant=InternalParameters  NCopyVariant=Disabled  FilterICVariant=InternalICsFilter  IntegratorICVariant=InternalICs  ExternalResetVariant=Disabled  TRSumVariant=Passthrough  SumFdbkVariant=Disabled  SumVariant=Sum_PID  TsampFilterVariant=InternalTs  TsampNgainVariant=Passthrough  TsampIntegralVariant=Passthrough  ExternalSaturationOutDataTypeStr=Inherit: Same as second input
  Saturation{,5..7} (4 alike) : Saturate  UpperLimit=50  LowerLimit=-50
  Saturation{1..4} (4 alike) : Saturate  UpperLimit=50  LowerLimit=0
  Sum{,1..7} (8 alike) : Sum  Inputs=-+|
  Out1 : Outport
  wires:
  In1/1 -> Demux/1
  Demux/1 -> Sum/2
  Sum/1 -> PID Controller5/1
  Constant/1 -> Sum/1
  PID Controller5/1 -> Saturation/1
  Mux/1 -> Out1/1
  Saturation/1 -> Mux/1
  Saturation1/1 -> Mux/5
  Sum3/1 -> PID Controller1/1
  PID Controller1/1 -> Saturation1/1
  Demux/5 -> Sum3/2
  Constant1/1 -> Sum3/1
  Demux/6 -> Sum2/2
  Constant4/1 -> Sum2/1
  PID Controller3/1 -> Saturation4/1
  Saturation4/1 -> Mux/6
  Sum2/1 -> PID Controller3/1
  PID Controller6/1 -> Saturation5/1
  Constant5/1 -> Sum5/1
  Demux/2 -> Sum5/2
  Sum5/1 -> PID Controller6/1
  PID Controller7/1 -> Saturation6/1
  Constant6/1 -> Sum6/1
  Saturation6/1 -> Mux/3
  Demux/3 -> Sum6/2
  Sum6/1 -> PID Controller7/1
  Sum7/1 -> PID Controller8/1
  PID Controller8/1 -> Saturation7/1
  Demux/4 -> Sum7/2
  Constant7/1 -> Sum7/1
  Saturation7/1 -> Mux/4
  Saturation5/1 -> Mux/2
  Sum1/1 -> PID Controller2/1
  Demux/8 -> Sum1/2
  PID Controller2/1 -> Saturation2/1
  Constant2/1 -> Sum1/1
  Sum4/1 -> PID Controller4/1
  Demux/7 -> Sum4/2
  PID Controller4/1 -> Saturation3/1
  Constant3/1 -> Sum4/1
  Saturation3/1 -> Mux/7
  Saturation2/1 -> Mux/8

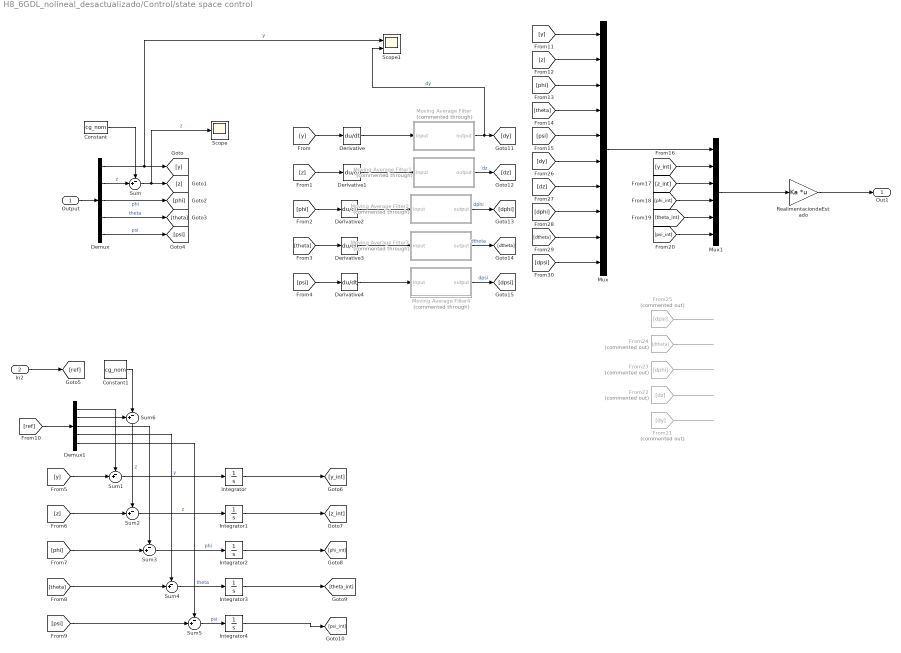
== system H8_6GDL_nolineal_desactualizado/Control/state space control ==
  Output : Inport
  In2 : Inport  Port=2
  Constant : Constant  Value=cg_nom
  Constant1 : Constant  Value=cg_nom
  Demux : Demux  Outputs=5
  Demux1 : Demux  Outputs=5
  Derivative{,1..4} (5 alike) : Derivative
  From21 : From  Commented=on  GotoTag=dy
  From22 : From  Commented=on  GotoTag=dz
  From23 : From  Commented=on  GotoTag=dphi
  From24 : From  Commented=on  GotoTag=dtheta
  From25 : From  Commented=on  GotoTag=dpsi
  Integrator{,1..4} (5 alike) : Integrator
  Moving Average Filter : Subsystem  Commented=through  mask{M=4, fs=-1}
      mask prompts: M "Orden del filtro (M)"; fs "Frecuencia de muestreo (fs)"
  Moving Average Filter1 : Subsystem  Commented=through  mask{M=4, fs=-1}
      mask prompts: M "Orden del filtro (M)"; fs "Frecuencia de muestreo (fs)"
  Moving Average Filter2 : Subsystem  Commented=through  mask{M=4, fs=-1}
      mask prompts: M "Orden del filtro (M)"; fs "Frecuencia de muestreo (fs)"
  Moving Average Filter3 : Subsystem  Commented=through  mask{M=4, fs=-1}
      mask prompts: M "Orden del filtro (M)"; fs "Frecuencia de muestreo (fs)"
  Moving Average Filter4 : Subsystem  Commented=through  mask{M=4, fs=-1}
      mask prompts: M "Orden del filtro (M)"; fs "Frecuencia de muestreo (fs)"
  Mux : Mux  Inputs=10
  Mux1 : Mux  Inputs=6
  RealimentaciondeEstado : Gain  Gain=Ka  Multiplication=Matrix(K*u)
  Scope : Scope
  Scope1 : Scope  NumInputPorts=2
  Sum{,1..5} (6 alike) : Sum  Inputs=-+|
  Sum6 : Sum  Inputs=+-|
  Out1 : Outport
  wires:
  Output/1 -> Demux/1
  Derivative/1 -> Moving Average Filter/1(input)
  Derivative1/1 -> Moving Average Filter1/1(input)
  Derivative2/1 -> Moving Average Filter2/1(input)
  Derivative3/1 -> Moving Average Filter3/1(input)
  Derivative4/1 -> Moving Average Filter4/1(input)
  Mux/1 -> Mux1/1
  Demux/1 -> Scope1/1, [y]  "y"
  Constant/1 -> Sum/1
  Sum/1 -> Scope/1, [z]  "z"
  Demux/2 -> Sum/2  "z"
  Demux/3 -> [phi]  "phi"
  Demux/4 -> [theta]  "theta"
  Demux/5 -> [psi]  "psi"
  [psi] -> Derivative4/1
  [theta] -> Derivative3/1
  [phi] -> Derivative2/1
  [z] -> Derivative1/1
  [y] -> Derivative/1
  In2/1 -> [ref]
  [ref] -> Demux1/1
  [y] -> Sum1/2
  [z] -> Sum2/2
  [phi] -> Sum3/2
  [theta] -> Sum4/2
  [psi] -> Sum5/2
  Demux1/1 -> Sum1/1
  Demux1/3 -> Sum3/1
  Demux1/4 -> Sum4/1
  Demux1/5 -> Sum5/1
  Sum1/1 -> Integrator/1  "y"
  Sum5/1 -> Integrator4/1  "psi"
  Sum4/1 -> Integrator3/1  "theta"
  Sum3/1 -> Integrator2/1  "phi"
  Sum2/1 -> Integrator1/1  "z"
  [y] -> Mux/1
  [z] -> Mux/2
  [phi] -> Mux/3
  [theta] -> Mux/4
  [psi] -> Mux/5
  Integrator/1 -> [y_int]
  Integrator1/1 -> [z_int]
  Integrator2/1 -> [phi_int]
  Integrator3/1 -> [theta_int]
  Moving Average Filter/1(output) -> Scope1/2, [dy]  "dy"
  Moving Average Filter1/1(output) -> [dz]  "dz"
  Moving Average Filter2/1(output) -> [dphi]  "dphi"
  Moving Average Filter4/1(output) -> [dpsi]  "dpsi"
  Moving Average Filter3/1(output) -> [dtheta]  "dtheta"
  [y_int] -> Mux1/2
  [psi_int] -> Mux1/6
  [theta_int] -> Mux1/5
  [phi_int] -> Mux1/4
  [z_int] -> Mux1/3
  Mux1/1 -> RealimentaciondeEstado/1
  Constant1/1 -> Sum6/2
  Demux1/2 -> Sum6/1
  Sum6/1 -> Sum2/1  "z"
  Integrator4/1 -> [psi_int]
  [dtheta] -> Mux/9
  [dy] -> Mux/6
  [dz] -> Mux/7
  [dpsi] -> Mux/10
  [dphi] -> Mux/8
  From23/1 -> ?
  From24/1 -> ?
  From22/1 -> ?
  From21/1 -> ?
  From25/1 -> ?
  RealimentaciondeEstado/1 -> Out1/1

== system H8_6GDL_nolineal_desactualizado/EMS/RL ==
  target voltage : Inport
  airgap : Inport  Port=2
  temperature : Inport  Port=3
  2-D Lookup Table : Lookup_n-D  BreakpointsForDimension1=ems.Airgap  BreakpointsForDimension2=ems.Flux_Current(2:55)  Table=ems.Inductance  InternalRulePriority=Speed  RndMeth=Simplest
      settings: InputPortMap=u0,u1
  Abs : Abs  SaturateOnIntegerOverflow=off
  Add : Sum  Inputs=+-
  Delay{,1..3} (4 alike) : Delay  DelayLength=1
  Divide : Product  Inputs=*/
  Divide1 : Product  Inputs=*/
  Divide2 : Product  Inputs=*/
  Integrator1 : Integrator
  Subsystem : Subsystem
  to mm : Gain  Gain=1000
  current : Outport
  wires:
  airgap/1 -> to mm/1
  Divide/1 -> Integrator1/1
  Add/1 -> Divide/1
  Integrator1/1 -> Abs/1, current/1, Delay3/1, Add/2  "current applied"
  2-D Lookup Table/1 -> Divide2/1  "L"
  target voltage/1 -> Divide1/1
  temperature/1 -> Delay2/1
  Divide1/1 -> Add/1
  Subsystem/1(R) -> Divide2/2, Divide1/2  "R"
  Delay3/1 -> Subsystem/1(Current)
  Delay2/1 -> Subsystem/2(Temperature)
  Divide2/1 -> Divide/2
  Delay1/1 -> 2-D Lookup Table/2
  Delay/1 -> 2-D Lookup Table/1
  Abs/1 -> Delay1/1
  to mm/1 -> Delay/1

== system H8_6GDL_nolineal_desactualizado/EMS/RL1 ==
  target voltage : Inport
  airgap : Inport  Port=2
  temperature : Inport  Port=3
  2-D Lookup Table : Lookup_n-D  BreakpointsForDimension1=ems.Airgap  BreakpointsForDimension2=ems.Flux_Current(2:55)  Table=ems.Inductance  InternalRulePriority=Speed  RndMeth=Simplest
      settings: InputPortMap=u0,u1
  Abs : Abs  SaturateOnIntegerOverflow=off
  Add : Sum  Inputs=+-
  Delay{,1..3} (4 alike) : Delay  DelayLength=1
  Divide : Product  Inputs=*/
  Divide1 : Product  Inputs=*/
  Divide2 : Product  Inputs=*/
  Integrator1 : Integrator
  Subsystem : Subsystem
  to mm : Gain  Gain=1000
  current : Outport
  wires:
  airgap/1 -> to mm/1
  Divide/1 -> Integrator1/1
  Add/1 -> Divide/1
  Integrator1/1 -> Abs/1, current/1, Delay3/1, Add/2  "current applied"
  2-D Lookup Table/1 -> Divide2/1  "L"
  target voltage/1 -> Divide1/1
  temperature/1 -> Delay2/1
  Divide1/1 -> Add/1
  Subsystem/1(R) -> Divide2/2, Divide1/2  "R"
  Delay3/1 -> Subsystem/1(Current)
  Delay2/1 -> Subsystem/2(Temperature)
  Divide2/1 -> Divide/2
  Delay1/1 -> 2-D Lookup Table/2
  Delay/1 -> 2-D Lookup Table/1
  Abs/1 -> Delay1/1
  to mm/1 -> Delay/1

== system H8_6GDL_nolineal_desactualizado/EMS/RL2 ==
  target voltage : Inport
  airgap : Inport  Port=2
  temperature : Inport  Port=3
  2-D Lookup Table : Lookup_n-D  BreakpointsForDimension1=ems.Airgap  BreakpointsForDimension2=ems.Flux_Current(2:55)  Table=ems.Inductance  InternalRulePriority=Speed  RndMeth=Simplest
      settings: InputPortMap=u0,u1
  Abs : Abs  SaturateOnIntegerOverflow=off
  Add : Sum  Inputs=+-
  Delay{,1..3} (4 alike) : Delay  DelayLength=1
  Divide : Product  Inputs=*/
  Divide1 : Product  Inputs=*/
  Divide2 : Product  Inputs=*/
  Integrator1 : Integrator
  Subsystem : Subsystem
  to mm : Gain  Gain=1000
  current : Outport
  wires:
  airgap/1 -> to mm/1
  Divide/1 -> Integrator1/1
  Add/1 -> Divide/1
  Integrator1/1 -> Abs/1, current/1, Delay3/1, Add/2  "current applied"
  2-D Lookup Table/1 -> Divide2/1  "L"
  target voltage/1 -> Divide1/1
  temperature/1 -> Delay2/1
  Divide1/1 -> Add/1
  Subsystem/1(R) -> Divide2/2, Divide1/2  "R"
  Delay3/1 -> Subsystem/1(Current)
  Delay2/1 -> Subsystem/2(Temperature)
  Divide2/1 -> Divide/2
  Delay1/1 -> 2-D Lookup Table/2
  Delay/1 -> 2-D Lookup Table/1
  Abs/1 -> Delay1/1
  to mm/1 -> Delay/1

== system H8_6GDL_nolineal_desactualizado/EMS/RL3 ==
  target voltage : Inport
  airgap : Inport  Port=2
  temperature : Inport  Port=3
  2-D Lookup Table : Lookup_n-D  BreakpointsForDimension1=ems.Airgap  BreakpointsForDimension2=ems.Flux_Current(2:55)  Table=ems.Inductance  InternalRulePriority=Speed  RndMeth=Simplest
      settings: InputPortMap=u0,u1
  Abs : Abs  SaturateOnIntegerOverflow=off
  Add : Sum  Inputs=+-
  Delay{,1..3} (4 alike) : Delay  DelayLength=1
  Divide : Product  Inputs=*/
  Divide1 : Product  Inputs=*/
  Divide2 : Product  Inputs=*/
  Integrator1 : Integrator
  Subsystem : Subsystem
  to mm : Gain  Gain=1000
  current : Outport
  wires:
  airgap/1 -> to mm/1
  Divide/1 -> Integrator1/1
  Add/1 -> Divide/1
  Integrator1/1 -> Abs/1, current/1, Delay3/1, Add/2  "current applied"
  2-D Lookup Table/1 -> Divide2/1  "L"
  target voltage/1 -> Divide1/1
  temperature/1 -> Delay2/1
  Divide1/1 -> Add/1
  Subsystem/1(R) -> Divide2/2, Divide1/2  "R"
  Delay3/1 -> Subsystem/1(Current)
  Delay2/1 -> Subsystem/2(Temperature)
  Divide2/1 -> Divide/2
  Delay1/1 -> 2-D Lookup Table/2
  Delay/1 -> 2-D Lookup Table/1
  Abs/1 -> Delay1/1
  to mm/1 -> Delay/1

== system H8_6GDL_nolineal_desactualizado/EMS/Subsystem1 ==
  current5 : Inport
  Constant : Constant  Value=0
  Constant2 : Constant  Value=50
  Switch : Switch  Criteria=u2 > Threshold  SaturateOnIntegerOverflow=off  InputSameDT=off
  Switch1 : Switch  Criteria=u2 > Threshold  Threshold=50  SaturateOnIntegerOverflow=off  InputSameDT=off
  Out1 : Outport
  wires:
  current5/1 -> Switch/1, Switch/2
  Switch1/1 -> Out1/1
  Switch/1 -> Switch1/3, Switch1/2
  Constant/1 -> Switch/3
  Constant2/1 -> Switch1/1

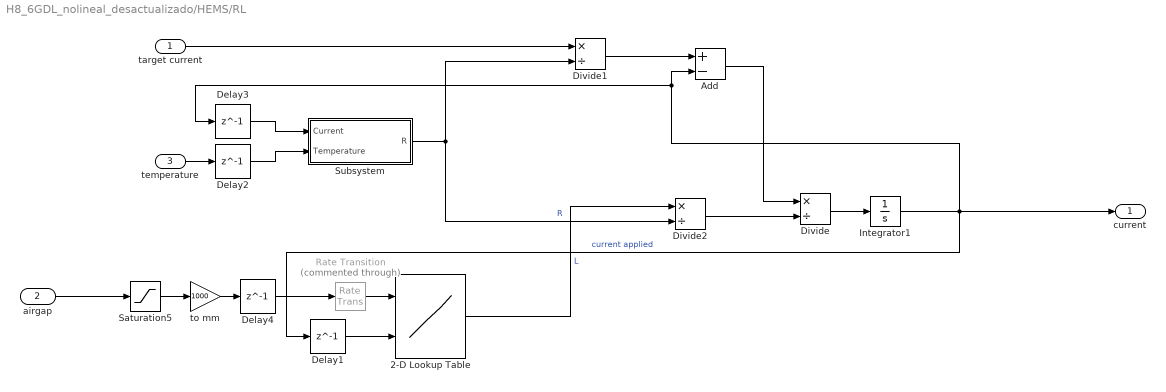
== system H8_6GDL_nolineal_desactualizado/HEMS/RL ==
  target current : Inport
  airgap : Inport  Port=2
  temperature : Inport  Port=3
  2-D Lookup Table : Lookup_n-D  BreakpointsForDimension1=hems.Airgap  BreakpointsForDimension2=hems.Current(2:110)  Table=hems.Inductance  InternalRulePriority=Speed  RndMeth=Simplest
      settings: InputPortMap=u0,u1
  Add : Sum  Inputs=+-
  Delay{1..4} (4 alike) : Delay  DelayLength=1
  Divide : Product  Inputs=*/
  Divide1 : Product  Inputs=*/
  Divide2 : Product  Inputs=*/
  Integrator1 : Integrator
  Rate Transition : RateTransition  Commented=through
  Saturation5 : Saturate  UpperLimit=0.0225  LowerLimit=0.01
  Subsystem : Subsystem
  to mm : Gain  Gain=1000
  current : Outport
  wires:
  airgap/1 -> Saturation5/1
  Divide/1 -> Integrator1/1
  Add/1 -> Divide/1
  Integrator1/1 -> Delay1/1, current/1, Delay3/1, Add/2  "current applied"
  2-D Lookup Table/1 -> Divide2/1  "L"
  target current/1 -> Divide1/1
  temperature/1 -> Delay2/1
  Divide1/1 -> Add/1
  Subsystem/1(R) -> Divide2/2, Divide1/2  "R"
  Delay3/1 -> Subsystem/1(Current)
  Delay2/1 -> Subsystem/2(Temperature)
  Divide2/1 -> Divide/2
  Delay1/1 -> 2-D Lookup Table/2
  Rate Transition/1 -> 2-D Lookup Table/1
  Saturation5/1 -> to mm/1
  to mm/1 -> Delay4/1
  Delay4/1 -> Rate Transition/1

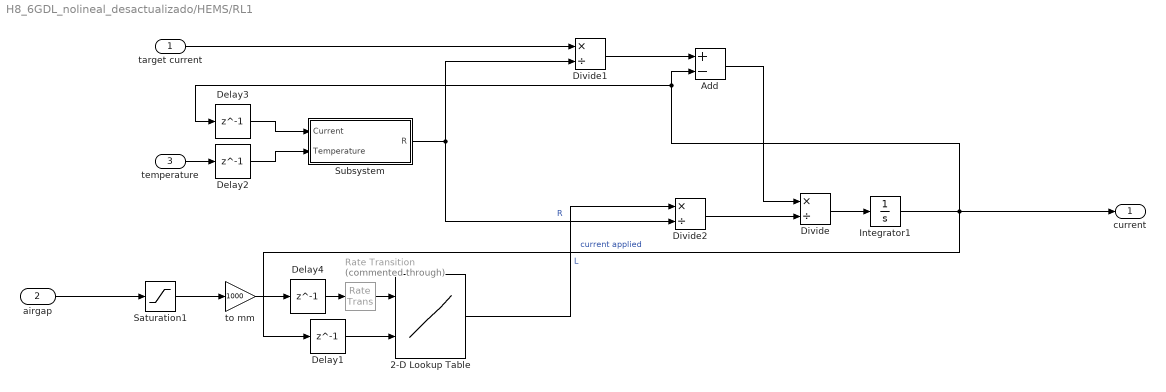
== system H8_6GDL_nolineal_desactualizado/HEMS/RL1 ==
  target current : Inport
  airgap : Inport  Port=2
  temperature : Inport  Port=3
  2-D Lookup Table : Lookup_n-D  BreakpointsForDimension1=hems.Airgap  BreakpointsForDimension2=hems.Current(2:110)  Table=hems.Inductance  InternalRulePriority=Speed  RndMeth=Simplest
      settings: InputPortMap=u0,u1
  Add : Sum  Inputs=+-
  Delay{1..4} (4 alike) : Delay  DelayLength=1
  Divide : Product  Inputs=*/
  Divide1 : Product  Inputs=*/
  Divide2 : Product  Inputs=*/
  Integrator1 : Integrator
  Rate Transition : RateTransition  Commented=through
  Saturation1 : Saturate  UpperLimit=0.0225  LowerLimit=0.01
  Subsystem : Subsystem
  to mm : Gain  Gain=1000
  current : Outport
  wires:
  airgap/1 -> Saturation1/1
  Divide/1 -> Integrator1/1
  Add/1 -> Divide/1
  Integrator1/1 -> Delay1/1, current/1, Delay3/1, Add/2  "current applied"
  2-D Lookup Table/1 -> Divide2/1  "L"
  target current/1 -> Divide1/1
  temperature/1 -> Delay2/1
  Divide1/1 -> Add/1
  Subsystem/1(R) -> Divide2/2, Divide1/2  "R"
  Delay3/1 -> Subsystem/1(Current)
  Delay2/1 -> Subsystem/2(Temperature)
  Divide2/1 -> Divide/2
  Delay1/1 -> 2-D Lookup Table/2
  Rate Transition/1 -> 2-D Lookup Table/1
  Saturation1/1 -> to mm/1
  to mm/1 -> Delay4/1
  Delay4/1 -> Rate Transition/1

== system H8_6GDL_nolineal_desactualizado/HEMS/RL2 ==
  target current : Inport
  airgap : Inport  Port=2
  temperature : Inport  Port=3
  2-D Lookup Table : Lookup_n-D  BreakpointsForDimension1=hems.Airgap  BreakpointsForDimension2=hems.Current(2:110)  Table=hems.Inductance  InternalRulePriority=Speed  RndMeth=Simplest
      settings: InputPortMap=u0,u1
  Add : Sum  Inputs=+-
  Delay{1..4} (4 alike) : Delay  DelayLength=1
  Divide : Product  Inputs=*/
  Divide1 : Product  Inputs=*/
  Divide2 : Product  Inputs=*/
  Integrator1 : Integrator
  Rate Transition : RateTransition  Commented=through
  Saturation5 : Saturate  UpperLimit=0.0225  LowerLimit=0.01
  Subsystem : Subsystem
  to mm : Gain  Gain=1000
  current : Outport
  wires:
  airgap/1 -> Saturation5/1
  Divide/1 -> Integrator1/1
  Add/1 -> Divide/1
  Integrator1/1 -> Delay1/1, current/1, Delay3/1, Add/2  "current applied"
  2-D Lookup Table/1 -> Divide2/1  "L"
  target current/1 -> Divide1/1
  temperature/1 -> Delay2/1
  Divide1/1 -> Add/1
  Subsystem/1(R) -> Divide2/2, Divide1/2  "R"
  Delay3/1 -> Subsystem/1(Current)
  Delay2/1 -> Subsystem/2(Temperature)
  Divide2/1 -> Divide/2
  Delay1/1 -> 2-D Lookup Table/2
  Rate Transition/1 -> 2-D Lookup Table/1
  Saturation5/1 -> to mm/1
  to mm/1 -> Delay4/1
  Delay4/1 -> Rate Transition/1

== system H8_6GDL_nolineal_desactualizado/HEMS/RL3 ==
  target current : Inport
  airgap : Inport  Port=2
  temperature : Inport  Port=3
  2-D Lookup Table : Lookup_n-D  BreakpointsForDimension1=hems.Airgap  BreakpointsForDimension2=hems.Current(2:110)  Table=hems.Inductance  InternalRulePriority=Speed  RndMeth=Simplest
      settings: InputPortMap=u0,u1
  Add : Sum  Inputs=+-
  Delay{1..4} (4 alike) : Delay  DelayLength=1
  Divide : Product  Inputs=*/
  Divide1 : Product  Inputs=*/
  Divide2 : Product  Inputs=*/
  Integrator1 : Integrator
  Rate Transition : RateTransition  Commented=through
  Saturation5 : Saturate  UpperLimit=0.0225  LowerLimit=0.01
  Subsystem : Subsystem
  to mm : Gain  Gain=1000
  current : Outport
  wires:
  airgap/1 -> Saturation5/1
  Divide/1 -> Integrator1/1
  Add/1 -> Divide/1
  Integrator1/1 -> Delay1/1, current/1, Delay3/1, Add/2  "current applied"
  2-D Lookup Table/1 -> Divide2/1  "L"
  target current/1 -> Divide1/1
  temperature/1 -> Delay2/1
  Divide1/1 -> Add/1
  Subsystem/1(R) -> Divide2/2, Divide1/2  "R"
  Delay3/1 -> Subsystem/1(Current)
  Delay2/1 -> Subsystem/2(Temperature)
  Divide2/1 -> Divide/2
  Delay1/1 -> 2-D Lookup Table/2
  Rate Transition/1 -> 2-D Lookup Table/1
  Saturation5/1 -> to mm/1
  to mm/1 -> Delay4/1
  Delay4/1 -> Rate Transition/1
